simulink library "lib_header"  (R2021b)
settings: Solver=VariableStepAuto  StartTime=0.0  StopTime=10.0  RelTol=1e-3
libraries: slrealtimeutilitieslib x1
settings Model: Creator=jiw19031  LastModifiedBy=jiw19031

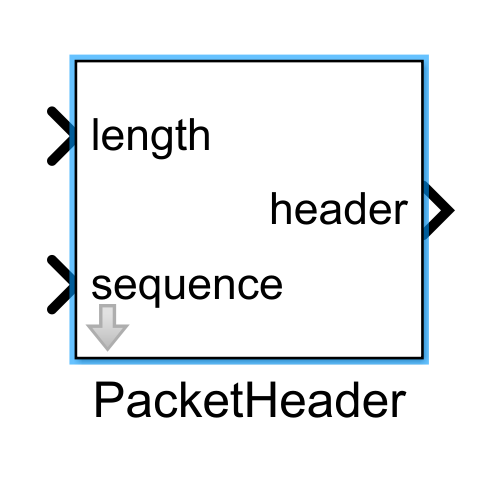
[thumbnail: Simulink's stored preview of the top-level diagram]
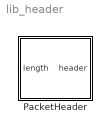
== system lib_header ==
  PacketHeader : Subsystem  mask{src=0, dst=0, pkt_type=0, pkt_priority=0, service=0, flag=0, option1=0, option2=0, subframe_num=0}
      mask prompts: pkt_type "Type"; pkt_priority "Priority"; subframe_num "SubframeNum"

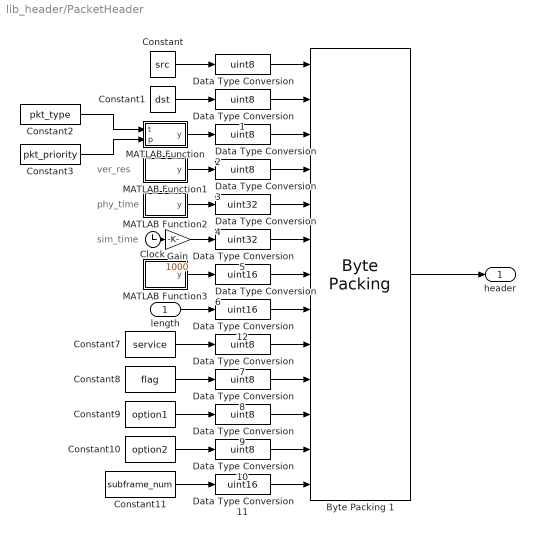
== system lib_header/PacketHeader ==
  note: sim_time
  note: phy_time
  note: ver_res
  length : Inport
  Byte Packing 1 : slrealtimeutilitieslib/Byte Packing  MaskPackedDataType=uint8  MaskUnpackedDataTypes={'uint8','uint8','uint8','uint8','uint32','uint32','uint16','uint16','uint8','uint8','uint8','uint8','uint16'}  MaskAlignment=1
  Clock : Clock
  Constant : Constant  Value=src
  Constant1 : Constant  Value=dst
  Constant10 : Constant  Value=option2
  Constant11 : Constant  Value=subframe_num
  Constant2 : Constant  Value=pkt_type
  Constant3 : Constant  Value=pkt_priority
  Constant7 : Constant  Value=service
  Constant8 : Constant  Value=flag
  Constant9 : Constant  Value=option1
  Data Type Conversion{,1..3,7..10} (8 alike) : DataTypeConversion  OutDataTypeStr=uint8
  Data Type Conversion11 : DataTypeConversion  OutDataTypeStr=uint16
  Data Type Conversion12 : DataTypeConversion  OutDataTypeStr=uint16
  Data Type Conversion4 : DataTypeConversion  OutDataTypeStr=uint32
  Data Type Conversion5 : DataTypeConversion  OutDataTypeStr=uint32
  Data Type Conversion6 : DataTypeConversion  OutDataTypeStr=uint16
  Gain : Gain  Gain=1000
  MATLAB Function : MATLAB Function  TreatAsAtomicUnit=on
  MATLAB Function1 : MATLAB Function  TreatAsAtomicUnit=on
  MATLAB Function2 : MATLAB Function  TreatAsAtomicUnit=on
  MATLAB Function3 : MATLAB Function  TreatAsAtomicUnit=on
  header : Outport
  wires:
  Byte Packing 1/1 -> header/1
  length/1 -> Data Type Conversion12/1
  Constant/1 -> Data Type Conversion/1
  Data Type Conversion/1 -> Byte Packing 1/1
  Data Type Conversion1/1 -> Byte Packing 1/2
  Constant1/1 -> Data Type Conversion1/1
  Constant2/1 -> MATLAB Function/1(t)
  Constant3/1 -> MATLAB Function/2(p)
  MATLAB Function/1(y) -> Data Type Conversion2/1
  Data Type Conversion2/1 -> Byte Packing 1/3
  MATLAB Function1/1(y) -> Data Type Conversion3/1
  Data Type Conversion3/1 -> Byte Packing 1/4
  Data Type Conversion4/1 -> Byte Packing 1/5
  MATLAB Function2/1(y) -> Data Type Conversion4/1
  Data Type Conversion5/1 -> Byte Packing 1/6
  Data Type Conversion6/1 -> Byte Packing 1/7
  Data Type Conversion7/1 -> Byte Packing 1/9
  Constant7/1 -> Data Type Conversion7/1
  Data Type Conversion8/1 -> Byte Packing 1/10
  Constant8/1 -> Data Type Conversion8/1
  Data Type Conversion9/1 -> Byte Packing 1/11
  Constant9/1 -> Data Type Conversion9/1
  Data Type Conversion10/1 -> Byte Packing 1/12
  Constant10/1 -> Data Type Conversion10/1
  Data Type Conversion11/1 -> Byte Packing 1/13
  Constant11/1 -> Data Type Conversion11/1
  Data Type Conversion12/1 -> Byte Packing 1/8
  Clock/1 -> Gain/1
  Gain/1 -> Data Type Conversion5/1
  MATLAB Function3/1(y) -> Data Type Conversion6/1

== matlab function lib_header/PacketHeader/MATLAB Function ==
  data: t input; y output; p input
function y = type_n_prior(t, p)
y = bitor( bitshift(t,4), p );

== matlab function lib_header/PacketHeader/MATLAB Function2 ==
  data: y output
function y = fcn()
y = uint32(posixtime(datetime('now')));

== matlab function lib_header/PacketHeader/MATLAB Function3 ==
  data: y output; Sequence data_store_memory
function y = fcn
%#codegen
global Sequence;
Sequence = Sequence + 1;
y = Sequence;

== matlab function lib_header/PacketHeader/MATLAB Function1 ==
  data: y output
function y = ver_n_res()
ver = 6;
res = 0;
y = bitor( bitshift(ver, 4), res );
